simulink model "GalvoModel_v161b"  (R2015a)
settings: Solver=ode45  SolverMode=SingleTasking  StartTime=0.0  StopTime=50e-3  RelTol=1e-3
values from neighbouring files (symbols this model uses):
  FS = 2.0E-6    [dataDict_galvoSystemParams.sldd]    (also in ddict.mat = 2e-06; modelInitScript.m = 2e-06)
  JR = 7.3E-9    [dataDict_galvoLSK040EF.sldd]    (also in dataDict_galvoMod6860.sldd = 6.0E-8
  KEL = 0.015    [dataDict_galvoLSK040EF.sldd]    (also in dataDict_galvoMod6860.sldd = 0.0093
  KEMF = 0.007    [dataDict_galvoLSK040EF.sldd]    (also in dataDict_galvoMod6860.sldd = 0.00974
  KFR = 4.0E-6    [dataDict_galvoLSK040EF.sldd]    (also in dataDict_galvoMod6860.sldd = 1.0E-10
  KPD : value not decoded    [dataDict_galvoSystemParams.sldd]
  KTBmess = 0.0    [dataDict_galvoLSK040EF.sldd]    (also in dataDict_galvoMod6860.sldd = 0.026642537473583278
  L = 0.0018    [dataDict_galvoLSK040EF.sldd]    (also in dataDict_galvoMod6860.sldd = 0.00016
  RL = 2.3    [dataDict_galvoLSK040EF.sldd]    (also in dataDict_galvoMod6860.sldd = 1.5
settings Model: DataDictionary=dataDict_galvoMod6860.sldd  Creator=mainster  LastModifiedBy=mainster
settings DataIOCC: SignalLoggingSaveFormat=ModelDataLogs
settings OptimizationCC: BlockReduction=off  BooleanDataType=off
settings DebuggingCC: SaveWithParameterizedLinksMsg=none  UnderspecifiedInitializationDetection=Classic  MergeDetectMultiDrivingBlocksExec=none  SignalResolutionControl=TryResolveAllWithWarning  MultiTaskDSMMsg=warning  MultiTaskCondExecSysMsg=none  ParameterPrecisionLossMsg=error  StateNameClashWarn=warning
settings HardwareCC: TargetUnknown=on

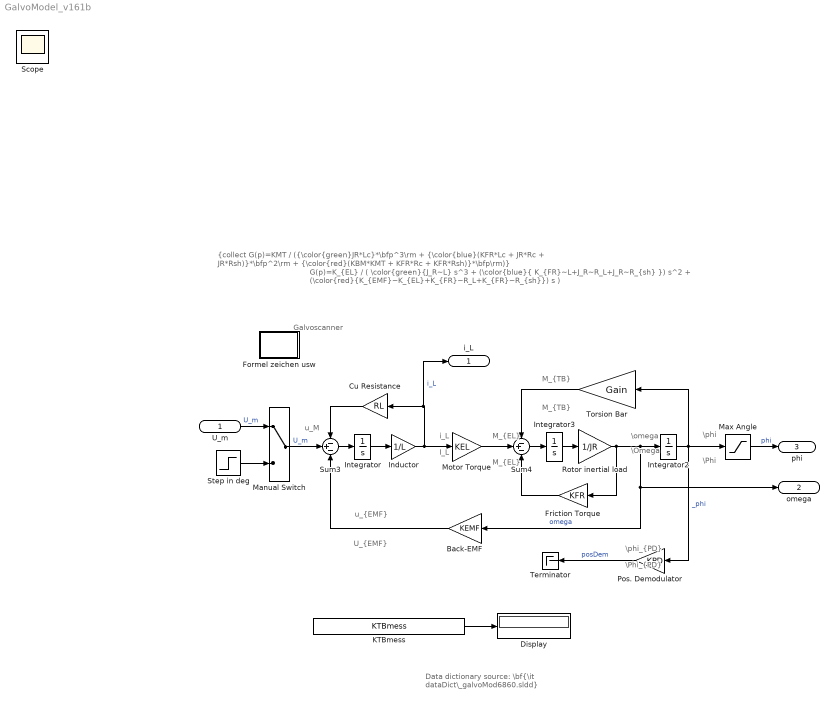
== system GalvoModel_v161b ==
  note: G(p)=K_{EL} / ( \color{green}{J_R~L} s^3 + (\color{blue}{ K_{FR}~L+J_R~R_L+J_R~R_{sh} }) s^2 + (\color{red}{K_{EMF}~K_{EL}+K_{FR}~R_L+K_{FR}~R_{sh}}) s )
  note: {collect G(p)=KMT / ({\color{green}JR*Lc}*\bfp^3\rm + {\color{blue}(KFR*Lc + JR*Rc + JR*Rsh)}*\bfp^2\rm + {\color{red}(KBM*KMT + KFR*Rc + KFR*Rsh)}*\bfp\rm)}
  note: Galvoscanner
  note: \Phi
  note: \phi
  note: u_M
  note: M_{EL}
  note: \omega
  note: i_L
  note: I_L
  note: M_{EL}
  note: \Omega
  note: M_{TB}
  note: M_{TB}
  note: u_{EMF}
  note: U_{EMF}
  note: \Phi_{PD}
  note: \phi_{PD}
  note: Data dictionary source:
      | \bf{\it dataDict\_galvoMod6860.sldd}
  U_m : Inport
  Back-EMF : Gain  Gain=KEMF
  Cu Resistance : Gain  Gain=RL
  Display : Display
  Formel zeichen usw : Subsystem
  Friction Torque : Gain  Gain=KFR
  Inductor : Gain  Gain=1/L
  Integrator : Integrator
  Integrator2 : Integrator
  Integrator3 : Integrator
  KTBmess : Constant  Value=KTBmess  SampleTime=FS
  Manual Switch : ManualSwitch
  Max Angle : Saturate  UpperLimit=20*pi/180  LowerLimit=-20*pi/180
      settings: AttributesFormatString=Max=%<UpperLimit>\nMin=%<LowerLimit>
  Motor Torque : Gain  Gain=KEL
  Pos. Demodulator : Gain  Gain=KPD
  Rotor inertial load : Gain  Gain=1/JR
  Step in deg : Step  Time=1e-3  SampleTime=FS  ZeroCross=off
      settings: AttributesFormatString=Ampl.: %<After>\ntime:%<Time>
  Sum3 : Sum  Inputs=-+-
  Sum4 : Sum  Inputs=-+-
  Terminator : Terminator
  Torsion Bar : Gain  Gain=Gain  ParamMin=ParamMin  ParamMax=ParamMax  OutMin=OutMin  OutMax=OutMax  SampleTime=SampleTime  mask{Gain=KTBmess, Multiplication=Element-wise(K.*u), SampleTime=-1, OutMin=[], OutMax=[], OutDataTypeStr=Inherit: Inherit via internal rule, LockScale=off, RndMeth=Floor, SaturateOnIntegerOverflow=off, ParamMin=[], ParamMax=[], ParamDataTypeStr=Inherit: Inherit via internal rule}
      mask prompts: Gain "Simulink:blkprm_prompts:GainGain"; Multiplication "Simulink:blkprm_prompts:GainMultiplication"; SampleTime "Simulink:blkprm_prompts:AllBlksSampleTime"; OutMin "Simulink:blkprm_prompts:OutputDesignMin"; OutMax "Simulink:blkprm_prompts:OutputDesignMax"; OutDataTypeStr "Simulink:blkprm_prompts:OUTPUT_UNIFIEDDATATYPE"; LockScale "Simulink:blkprm_prompts:LockScale"; RndMeth "Simulink:blkprm_prompts:SPP_RndMeth_ID"; SaturateOnIntegerOverflow "Simulink:blkprm_prompts:AllBlksSaturate"; ParamMin "Simulink:blkprm_prompts:ParameterDesignMin"; ParamMax "Simulink:blkprm_prompts:ParameterDesignMax"; ParamDataTypeStr "Simulink:blkprm_prompts:PARAMETER_UNIFIEDDATATYPE"
      mask TypeOptions Gain: Gain
      mask TypeOptions Multiplication: Multiplication
      mask TypeOptions SampleTime: SampleTime
      mask TypeOptions OutMin: OutMin
      mask TypeOptions OutMax: OutMax
      mask TypeOptions OutDataTypeStr: OutDataTypeStr
      mask TypeOptions LockScale: LockScale
      mask TypeOptions RndMeth: RndMeth
      mask TypeOptions SaturateOnIntegerOverflow: SaturateOnIntegerOverflow
      mask TypeOptions ParamMin: ParamMin
      mask TypeOptions ParamMax: ParamMax
      mask TypeOptions ParamDataTypeStr: ParamDataTypeStr
      mask Display:
      | ddo=Simulink.data.dictionary.open(get_param(gcs,'DataDictionary'));
      | dds=ddo.getSection('Design Data');
      | 
      | fprintf('KTB=\n%g', Gain);
  i_L : Outport
  omega : Outport  Port=2
  phi : Outport  Port=3
  Scope : Scope  NumInputPorts=5
      settings: ShowLegends=on  TimeRange=0.015  YMin=0~0~0~-5~-5  YMax=70~0.35~20~5~5  MaxDataPoints=7500
  wires:
  U_m/1 -> Manual Switch/1  "U_m"
  KTBmess/1 -> Display/1
  Max Angle/1 -> phi/1  "phi"
  Manual Switch/1 -> Sum3/2  "U_m"
  Step in deg/1 -> Manual Switch/2
  Back-EMF/1 -> Sum3/3
  Sum3/1 -> Integrator/1
  Cu Resistance/1 -> Sum3/1
  Integrator/1 -> Inductor/1
  Inductor/1 -> Motor Torque/1, i_L/1, Cu Resistance/1  "i_L"
  Motor Torque/1 -> Sum4/2
  Integrator2/1 -> Torsion Bar/1, Max Angle/1, Pos. Demodulator/1  "_phi"
  Sum4/1 -> Integrator3/1
  Integrator3/1 -> Rotor inertial load/1
  Friction Torque/1 -> Sum4/3
  Rotor inertial load/1 -> Friction Torque/1, omega/1, Back-EMF/1, Integrator2/1  "omega"
  Pos. Demodulator/1 -> Terminator/1  "posDem"
  Torsion Bar/1 -> Sum4/1

== system GalvoModel_v161b/Formel zeichen usw ==
  note: Te: 		electrical torque, gen. by coils		[Nm]
      |  Ic: 			coil current							[A]
      |  Tfr:		rotor dynamic friction torque 		[Nm]
      |  Trb:		torsion bar torque					[Nm]
      |  Tw:		angular momentum				[Nm*s]
      |  w:			angular velocity 					[rad/s]
      |  yrad:		angular position 					[rad]
      |  ydeg:		angular position 					[°]
      |  Ucci:		current controller input				[V]
      |  Ucco:		current controller output			[V]
      |  Ush:		shunt voltage						[V]
  note: balance of force: 	Te=Ttb+Tfr
      | 					Te - (Ttb+Tfr)=0  ->  no movement
      |
      |  integrate( 1 Nm )dt = 1 Nm*s
      |  (Nm*s)(kg*m²)⁻¹ = (N*s/kg)*m⁻¹ = m/(s*m) = rad
  note: L_{c  }	coil inductance 							[H]
      |  R_{c  }	coil resistance							[\Omega]
      |  R_{SH }	current shunt resistance				[\Omega]
      |  J_{R  }	rotor inertia 							[kg*m²]
      |  \color{red}K_{TB }	torsion bar torque const. 			[Nm/rad]
      |  \color{black}K_{BM }	back EMF const.							[V*s/rad]
      |  K_{FR }	rotor dyn. friction torque const.	[Nm*s/rad]
      |  K_{MT }	el. magnetic torque const.			[Nm/A]
  note: ranging factor [V/A]:
      | Eingangsspannungsbereich des
      | Stromreglers z.B.:
      | -5V...5V --> -20A...20A
      | Kcc = 0.25V/A
  note: Shunt factor:
      | Ksh = L_mon*Rsh
      |
      | eg: Rsh = 10mOhm
      |
      | --> Ksh = 250mV/A
      | max. shunt monitor
      | output Vswing:
      | 20A*Ksh = 5V
  note: INA225:
      | Gain:		Accuracy:		Bandwidth:
      | 25V/V		+-0.15%		250kHz
      | 50V/V		+-0.15%		?
      | 100V/V	+-0.20%		?
      | 200V/V	+-0.30%		?
